simulink model "VCU_Control_Test"  (R2026a)
settings: Solver=VariableStepAuto  StopTime=Motor_Torque_Data.Time(end)
settings Model: Creator=renil  LastModifiedBy=renil

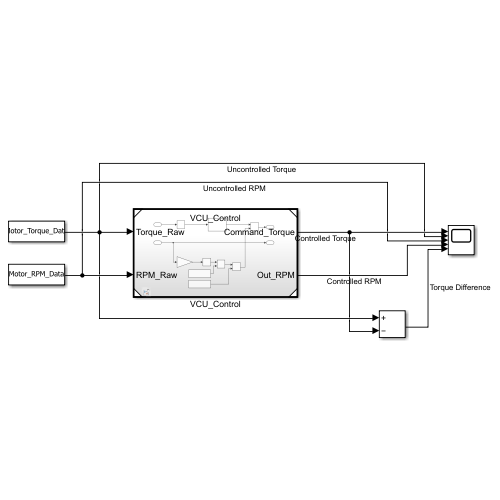
[thumbnail: Simulink's stored preview of the top-level diagram]
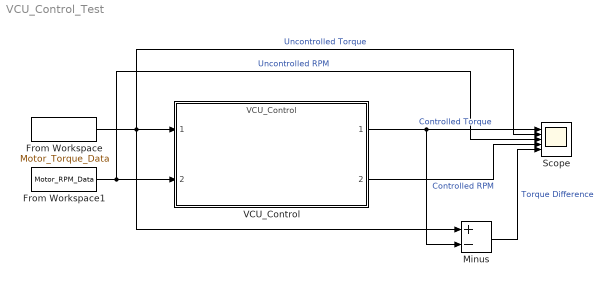
== system VCU_Control_Test ==
  From Workspace : FromWorkspace  VariableName=Motor_Torque_Data
  From Workspace1 : FromWorkspace  VariableName=Motor_RPM_Data
  Minus : Sum  Inputs=+-
  Scope : Scope  NumInputPorts=5
      settings: ActiveDisplayYMinimum=-435.59250304101397  ActiveDisplayYMaximum=795.56296439055677  DataLoggingVariableName=VCUScopeData
  VCU_Control : ModelReference  ModelNameDialog=VCU_Control.slx  SimulationMode=Normal  ModelReferenceVersion=1.7
  wires:
  From Workspace/1 -> Scope/2, VCU_Control/1, Minus/1  "Uncontrolled Torque"
  From Workspace1/1 -> Scope/3, VCU_Control/2  "Uncontrolled RPM"
  VCU_Control/1 -> Minus/2, Scope/1  "Controlled Torque"
  VCU_Control/2 -> Scope/4  "Controlled RPM"
  Minus/1 -> Scope/5  "Torque Difference"
